simulink model "ducted_fan"  (R2014a)
settings: Solver=ode45  StartTime=0.0  StopTime=10.0  RelTol=1e-3
undefined symbols (not defined in the file): DiscIntNeverNeededParam, ST
libraries: simulink_extras x15
settings Model: Creator=stefa  LastModifiedBy=stefa

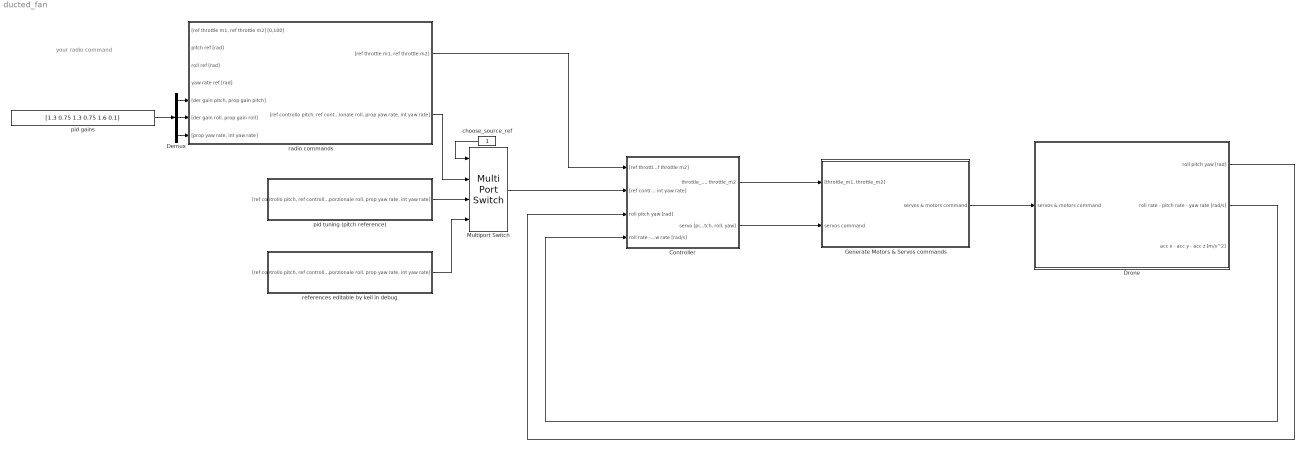
== system ducted_fan ==
  note: your radio command
  Controller : Subsystem
  Demux : Demux  Outputs=[2 2 2]
  Drone : Subsystem
  Generate Motors & Servos commands : Subsystem
  Multiport Switch : MultiPortSwitch
  choose_source_ref : Constant
  pid gains : Constant  Value=[1.3 0.75 1.3 0.75 1.6 0.1]
  pid tuning (pitch reference) : Subsystem
  radio commands : Subsystem
  references editable by keil in debug : Subsystem
  wires:
  Drone/1(roll pitch yaw [rad]) -> Controller/3(roll pitch yaw [rad])
  Drone/2(roll rate - pitch rate - yaw rate [rad/s]) -> Controller/4(roll rate - pitch rate - yaw rate [rad/s])
  Controller/2("servo [pitch, roll, yaw]") -> Generate Motors & Servos commands/2(servos command)
  Generate Motors & Servos commands/1(servos & motors command) -> Drone/1(servos & motors command)
  Controller/1("throttle_m1, throttle_m2") -> Generate Motors & Servos commands/1("[throttle_m1, throttle_m2]")
  choose_source_ref/1 -> Multiport Switch/1
  Multiport Switch/1 -> Controller/2("[ref controllo pitch, ref controllo roll, ref controllo yaw rate, guadagno derivativo pitch, guadagno proporzionale pitch, guadagno derivativo roll, guadagno proporzionale roll, prop yaw rate, int yaw rate]")
  radio commands/2("[ref controllo pitch, ref controllo roll, ref controllo yaw rate, guadagno derivativo pitch, guadagno proporzionale pitch, guadagno derivativo roll, guadagno proporzionale roll, prop yaw rate, int yaw rate]") -> Multiport Switch/2
  pid tuning (pitch reference)/1("[ref controllo pitch, ref controllo roll, ref controllo yaw rate, guadagno derivativo pitch, guadagno proporzionale pitch, guadagno derivativo roll, guadagno proporzionale roll, prop yaw rate, int yaw rate]") -> Multiport Switch/3
  references editable by keil in debug/1("[ref controllo pitch, ref controllo roll, ref controllo yaw rate, guadagno derivativo pitch, guadagno proporzionale pitch, guadagno derivativo roll, guadagno proporzionale roll, prop yaw rate, int yaw rate]") -> Multiport Switch/4
  radio commands/1("[ref throttle m1, ref throttle m2]") -> Controller/1("[ref throttle m1, ref throttle m2]")
  ? -> radio commands/1("[ref throttle m1, ref throttle m2] [0,100]")
  ? -> radio commands/2(pitch ref [rad])
  ? -> radio commands/3(roll ref [rad])
  ? -> radio commands/4(yaw rate ref [rad])
  Demux/2 -> radio commands/6("[der gain roll, prop gain roll]")
  Demux/1 -> radio commands/5("[der gain pitch, prop gain pitch]")
  Demux/3 -> radio commands/7("[prop yaw rate, int yaw rate]")
  pid gains/1 -> Demux/1

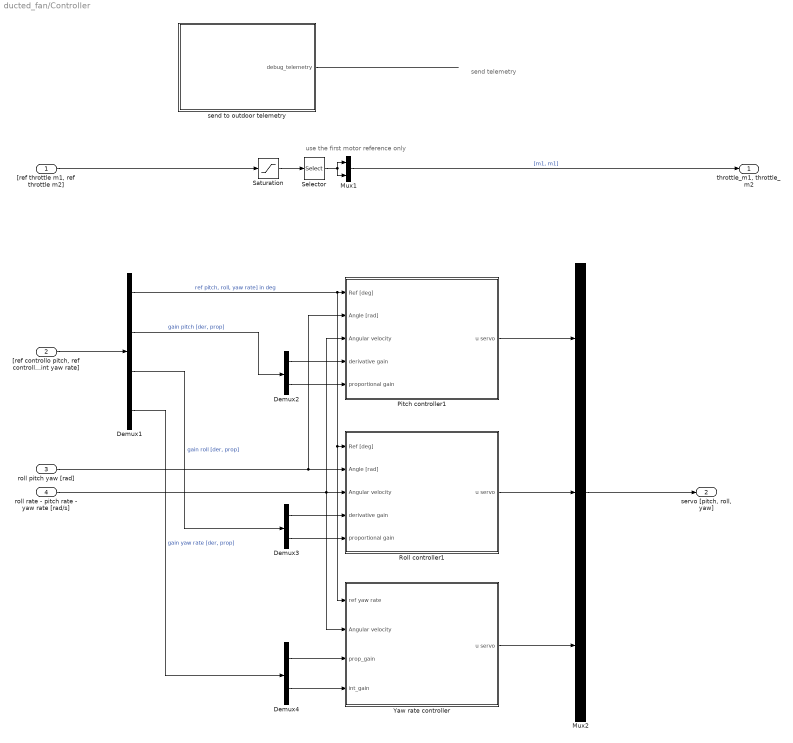
== system ducted_fan/Controller ==
  note: send telemetry
  note: use the first motor reference only
  "[ref throttle m1, ref throttle m2]" : Inport
  "[ref controllo pitch, ref controllo roll, ref controllo yaw rate, guadagno derivativo pitch, guadagno proporzionale pitch, guadagno derivativo roll, guadagno proporzionale roll, prop yaw rate, int yaw rate]" : Inport  Port=2
  roll pitch yaw [rad] : Inport  Port=3
  roll rate - pitch rate - yaw rate [rad/s] : Inport  Port=4
  Demux1 : Demux  Outputs=[3 2 2 2]
  Demux2 : Demux  Outputs=2
  Demux3 : Demux  Outputs=2
  Demux4 : Demux  Outputs=2
  Mux1 : Mux  Inputs=2
  Mux2 : Mux  Inputs=3
  Pitch controller1 : Subsystem
  Roll controller1 : Subsystem
  Saturation : Saturate  UpperLimit=100  LowerLimit=0
  Selector : Selector  InputPortWidth=2
  Yaw rate controller : Subsystem
  "send to outdoor telemetry " : Subsystem
  "throttle_m1, throttle_m2" : Outport
  "servo [pitch, roll, yaw]" : Outport  Port=2
  wires:
  Saturation/1 -> Selector/1
  Selector/1 -> Mux1/2, Mux1/1
  Mux1/1 -> "throttle_m1, throttle_m2"/1  "[m1, m1]"
  roll pitch yaw [rad]/1 -> Pitch controller1/2(Angle [rad]), Roll controller1/2(Angle [rad])
  roll rate - pitch rate - yaw rate [rad/s]/1 -> Pitch controller1/3(Angular velocity), Yaw rate controller/2(Angular velocity), Roll controller1/3(Angular velocity)
  Pitch controller1/1(u servo) -> Mux2/1
  Mux2/1 -> "servo [pitch, roll, yaw]"/1
  "[ref controllo pitch, ref controllo roll, ref controllo yaw rate, guadagno derivativo pitch, guadagno proporzionale pitch, guadagno derivativo roll, guadagno proporzionale roll, prop yaw rate, int yaw rate]"/1 -> Demux1/1
  Demux1/1 -> Yaw rate controller/1(ref yaw rate), Roll controller1/1(Ref [deg]), Pitch controller1/1(Ref [deg])  "ref pitch, roll, yaw rate] in deg"
  Roll controller1/1(u servo) -> Mux2/2
  Yaw rate controller/1(u servo) -> Mux2/3
  Demux1/2 -> Demux2/1  "gain pitch [der, prop]"
  Demux2/2 -> Pitch controller1/5(proportional gain)
  Demux2/1 -> Pitch controller1/4(derivative gain)
  Demux1/3 -> Demux3/1  "gain roll [der, prop]"
  Demux3/1 -> Roll controller1/4(derivative gain)
  Demux3/2 -> Roll controller1/5(proportional gain)
  Demux1/4 -> Demux4/1  "gain yaw rate [der, prop]"
  Demux4/1 -> Yaw rate controller/3(prop_gain)
  Demux4/2 -> Yaw rate controller/4(int_gain)
  "[ref throttle m1, ref throttle m2]"/1 -> Saturation/1
  "send to outdoor telemetry "/1(debug_telemetry) -> ?

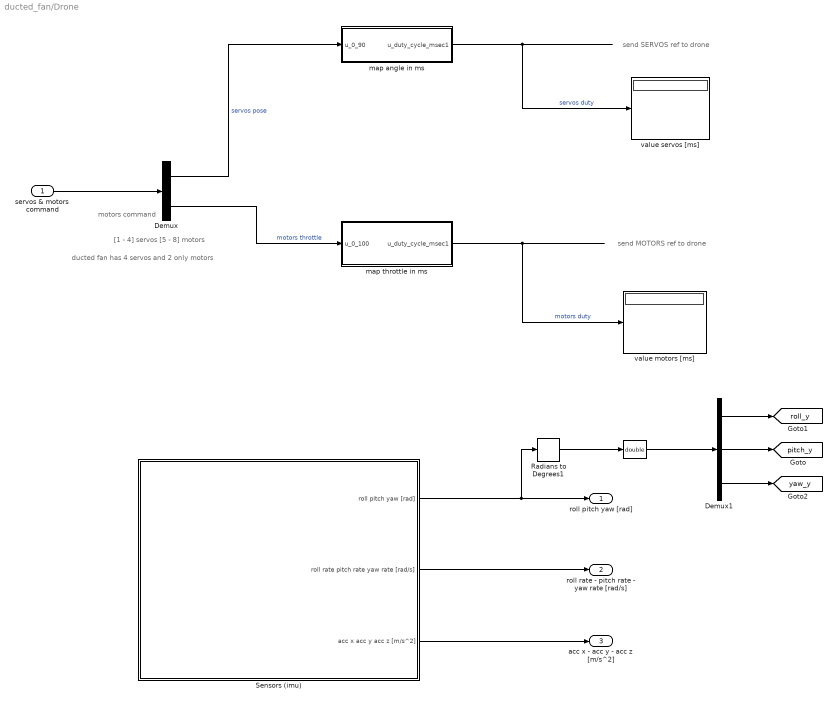
== system ducted_fan/Drone ==
  note: send SERVOS ref to drone
  note: ducted fan has 4 servos and 2 only motors
  note: [1 - 4] servos
      | [5 - 8] motors
  note: motors command
  note: send MOTORS ref to drone
  servos & motors command : Inport
  "  " : DataTypeConversion  OutDataTypeStr=double
  Demux : Demux  Outputs=[4 4]
  Demux1 : Demux  Outputs=3
  Radians to Degrees1 : simulink_extras/Transformations/Radians to Degrees
  Sensors (imu) : Subsystem
  map angle in ms : MATLAB Function  TreatAsAtomicUnit=on
  map throttle in ms : MATLAB Function  TreatAsAtomicUnit=on
  value motors [ms] : Display
  value servos [ms] : Display
  roll pitch yaw [rad] : Outport
  roll rate - pitch rate - yaw rate [rad/s] : Outport  Port=2
  acc x - acc y - acc z [m/s^2] : Outport  Port=3
  tag scope: pitch_y=global, roll_y=global, yaw_y=global
  wires:
  servos & motors command/1 -> Demux/1
  Demux/1 -> map angle in ms/1(u_0_90)  "servos pose"
  map throttle in ms/1(u_duty_cycle_msec1) -> value motors [ms]/1  "motors duty"
  map angle in ms/1(u_duty_cycle_msec1) -> value servos [ms]/1  "servos duty"
  Sensors (imu)/1(roll pitch yaw [rad]) -> Radians to Degrees1/1, roll pitch yaw [rad]/1
  Sensors (imu)/2(roll rate pitch rate yaw rate [rad/s]) -> roll rate - pitch rate - yaw rate [rad/s]/1
  Sensors (imu)/3(acc x acc y acc z [m/s^2]) -> acc x - acc y - acc z [m/s^2]/1
  Demux/2 -> map throttle in ms/1(u_0_100)  "motors throttle"
  Demux1/2 -> [pitch_y]
  Demux1/1 -> [roll_y]
  Radians to Degrees1/1 -> "  "/1
  "  "/1 -> Demux1/1
  Demux1/3 -> [yaw_y]

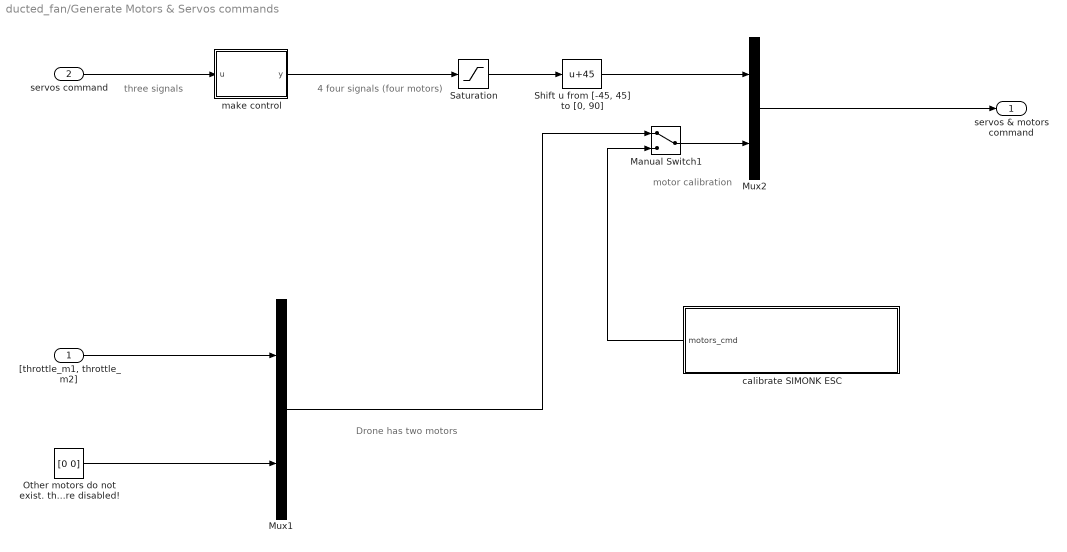
== system ducted_fan/Generate Motors & Servos commands ==
  note: 4 four signals (four motors)
  note: three signals
  note: Drone has two motors
  note: motor
      | calibration
  "[throttle_m1, throttle_m2]" : Inport
  servos command : Inport  Port=2
  Manual Switch1 : ManualSwitch
  Mux1 : Mux  Inputs=[2 2]
  Mux2 : Mux  Inputs=2
  Other motors do not exist. they are disabled! : Constant  Value=[0 0]
  Saturation : Saturate  UpperLimit=45  LowerLimit=-45
  "Shift u from [-45, 45] to [0, 90]" : Bias  Bias=45
  calibrate SIMONK ESC : Subsystem
  make control : MATLAB Function  TreatAsAtomicUnit=on
  servos & motors command : Outport
  wires:
  Mux2/1 -> servos & motors command/1
  Mux1/1 -> Manual Switch1/1
  calibrate SIMONK ESC/1(motors_cmd) -> Manual Switch1/2
  make control/1(y) -> Saturation/1
  Other motors do not exist. they are disabled!/1 -> Mux1/2
  Manual Switch1/1 -> Mux2/2
  servos command/1 -> make control/1(u)
  "[throttle_m1, throttle_m2]"/1 -> Mux1/1
  "Shift u from [-45, 45] to [0, 90]"/1 -> Mux2/1
  Saturation/1 -> "Shift u from [-45, 45] to [0, 90]"/1

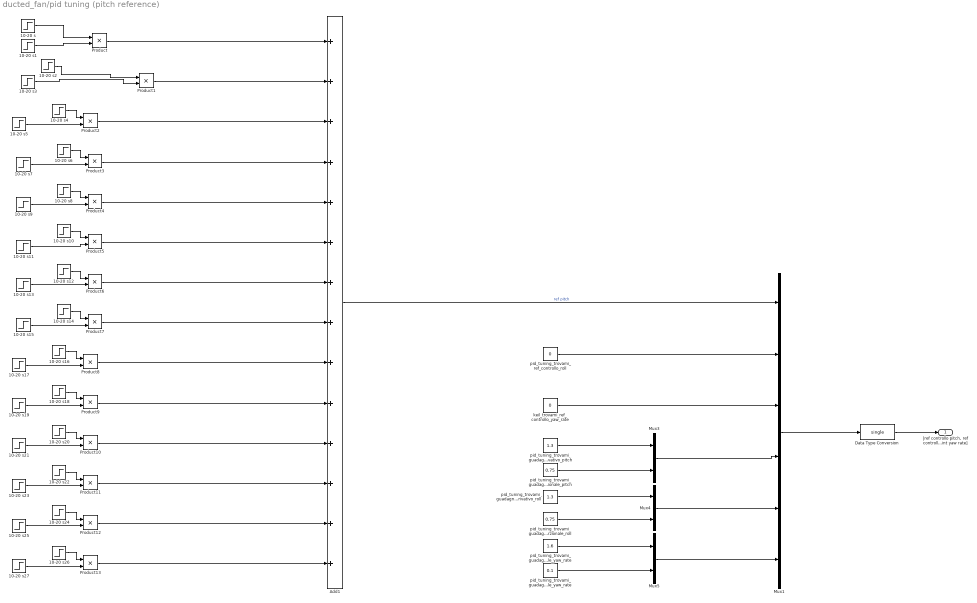
== system ducted_fan/pid tuning (pitch reference) ==
  10-20 s : Step  Time=20  After=10
  10-20 s1 : Step  Time=30  Before=1  After=0
  10-20 s10 : Step  Time=70  After=0
  10-20 s11 : Step  Time=80  Before=1  After=0
  10-20 s12 : Step  Time=80  After=-10
  10-20 s13 : Step  Time=90  Before=1  After=0
  10-20 s14 : Step  Time=90  After=0
  10-20 s15 : Step  Time=100  Before=1  After=0
  10-20 s16 : Step  Time=100  After=-20
  10-20 s17 : Step  Time=110  Before=1  After=0
  10-20 s18 : Step  Time=110  After=0
  10-20 s19 : Step  Time=120  Before=1  After=0
  10-20 s2 : Step  Time=30  After=0
  10-20 s20 : Step  Time=120  After=-30
  10-20 s21 : Step  Time=130  Before=1  After=0
  10-20 s22 : Step  Time=130  After=0
  10-20 s23 : Step  Time=140  Before=1  After=0
  10-20 s24 : Step  Time=140  After=40
  10-20 s25 : Step  Time=150  Before=1  After=0
  10-20 s26 : Step  Time=150  After=-40
  10-20 s27 : Step  Time=160  Before=1  After=0
  10-20 s3 : Step  Time=40  Before=1  After=0
  10-20 s4 : Step  Time=40  After=20
  10-20 s5 : Step  Time=50  Before=1  After=0
  10-20 s6 : Step  Time=50  After=0
  10-20 s7 : Step  Time=60  Before=1  After=0
  10-20 s8 : Step  Time=60  After=30
  10-20 s9 : Step  Time=70  Before=1  After=0
  Add1 : Sum  Inputs=++++++++++++++
  Data Type Conversion : DataTypeConversion  OutDataTypeStr=single
  Mux1 : Mux  Inputs=6
  Mux3 : Mux  Inputs=2
  Mux4 : Mux  Inputs=2
  Mux5 : Mux  Inputs=2
  Product{,1..13} (14 alike) : Product
  keil_trovami_ref_controllo_yaw_rate : Constant  Value=0  OutDataTypeStr=double  SampleTime=-1
  pid_tuning_trovami_guadagno_derivativo_pitch : Constant  Value=1.3  SampleTime=-1
  pid_tuning_trovami_guadagno_derivativo_roll : Constant  Value=1.3  SampleTime=-1
  pid_tuning_trovami_guadagno_integrale_yaw_rate : Constant  Value=0.1  SampleTime=-1
  pid_tuning_trovami_guadagno_proporzionale_pitch : Constant  Value=0.75  SampleTime=-1
  pid_tuning_trovami_guadagno_proporzionale_roll : Constant  Value=0.75  SampleTime=-1
  pid_tuning_trovami_guadagno_proporzionale_yaw_rate : Constant  Value=1.6  SampleTime=-1
  pid_tuning_trovami_ref_controllo_roll : Constant  Value=0  SampleTime=-1
  "[ref controllo pitch, ref controllo roll, ref controllo yaw rate, guadagno derivativo pitch, guadagno proporzionale pitch, guadagno derivativo roll, guadagno proporzionale roll, prop yaw rate, int yaw rate]" : Outport
  wires:
  Mux1/1 -> Data Type Conversion/1
  pid_tuning_trovami_ref_controllo_roll/1 -> Mux1/2
  10-20 s/1 -> Product/1
  Product/1 -> Add1/1
  10-20 s1/1 -> Product/2
  10-20 s2/1 -> Product1/1
  Product1/1 -> Add1/2
  10-20 s3/1 -> Product1/2
  10-20 s4/1 -> Product2/1
  Product2/1 -> Add1/3
  10-20 s5/1 -> Product2/2
  10-20 s6/1 -> Product3/1
  10-20 s7/1 -> Product3/2
  Product3/1 -> Add1/4
  10-20 s8/1 -> Product4/1
  10-20 s9/1 -> Product4/2
  Product4/1 -> Add1/5
  10-20 s10/1 -> Product5/1
  10-20 s11/1 -> Product5/2
  Product5/1 -> Add1/6
  10-20 s12/1 -> Product6/1
  10-20 s13/1 -> Product6/2
  Product6/1 -> Add1/7
  10-20 s14/1 -> Product7/1
  10-20 s15/1 -> Product7/2
  Product7/1 -> Add1/8
  10-20 s16/1 -> Product8/1
  10-20 s17/1 -> Product8/2
  Product8/1 -> Add1/9
  10-20 s18/1 -> Product9/1
  10-20 s19/1 -> Product9/2
  Product9/1 -> Add1/10
  10-20 s20/1 -> Product10/1
  10-20 s21/1 -> Product10/2
  Product10/1 -> Add1/11
  10-20 s22/1 -> Product11/1
  10-20 s23/1 -> Product11/2
  Product11/1 -> Add1/12
  10-20 s24/1 -> Product12/1
  10-20 s25/1 -> Product12/2
  Product12/1 -> Add1/13
  10-20 s26/1 -> Product13/1
  10-20 s27/1 -> Product13/2
  Product13/1 -> Add1/14
  Add1/1 -> Mux1/1  "ref pitch"
  Data Type Conversion/1 -> "[ref controllo pitch, ref controllo roll, ref controllo yaw rate, guadagno derivativo pitch, guadagno proporzionale pitch, guadagno derivativo roll, guadagno proporzionale roll, prop yaw rate, int yaw rate]"/1
  pid_tuning_trovami_guadagno_derivativo_pitch/1 -> Mux3/1
  pid_tuning_trovami_guadagno_derivativo_roll/1 -> Mux4/1
  pid_tuning_trovami_guadagno_proporzionale_pitch/1 -> Mux3/2
  Mux3/1 -> Mux1/4
  pid_tuning_trovami_guadagno_proporzionale_roll/1 -> Mux4/2
  Mux4/1 -> Mux1/5
  pid_tuning_trovami_guadagno_proporzionale_yaw_rate/1 -> Mux5/1
  pid_tuning_trovami_guadagno_integrale_yaw_rate/1 -> Mux5/2
  Mux5/1 -> Mux1/6
  keil_trovami_ref_controllo_yaw_rate/1 -> Mux1/3

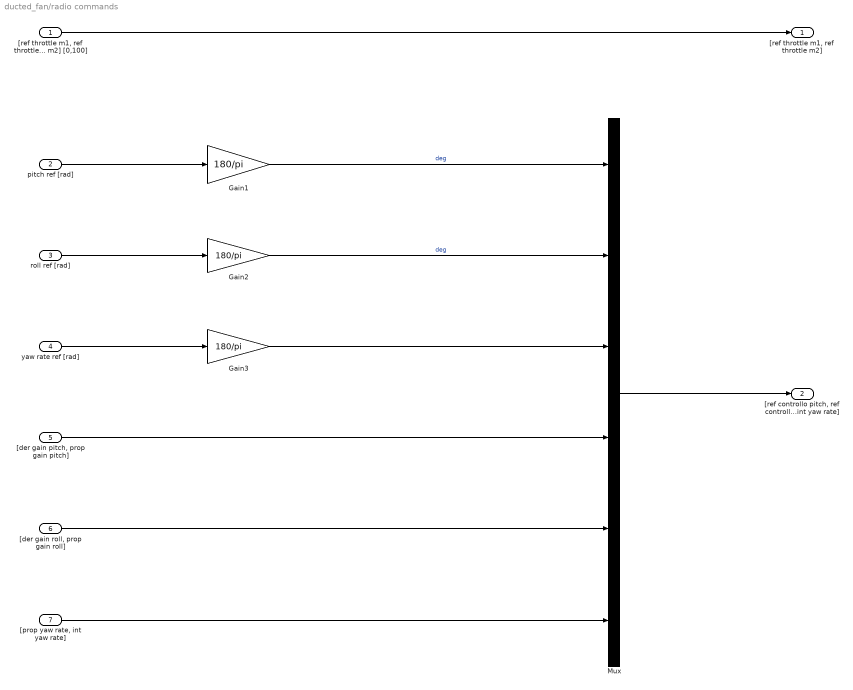
== system ducted_fan/radio commands ==
  "[ref throttle m1, ref throttle m2] [0,100]" : Inport
  pitch ref [rad] : Inport  Port=2
  roll ref [rad] : Inport  Port=3
  yaw rate ref [rad] : Inport  Port=4
  "[der gain pitch, prop gain pitch]" : Inport  Port=5
  "[der gain roll, prop gain roll]" : Inport  Port=6
  "[prop yaw rate, int yaw rate]" : Inport  Port=7
  Gain1 : Gain  Gain=180/pi
  Gain2 : Gain  Gain=180/pi
  Gain3 : Gain  Gain=180/pi
  Mux : Mux  Inputs=[1 1 1 2 2 2]
  "[ref throttle m1, ref throttle m2]" : Outport
  "[ref controllo pitch, ref controllo roll, ref controllo yaw rate, guadagno derivativo pitch, guadagno proporzionale pitch, guadagno derivativo roll, guadagno proporzionale roll, prop yaw rate, int yaw rate]" : Outport  Port=2
  wires:
  Mux/1 -> "[ref controllo pitch, ref controllo roll, ref controllo yaw rate, guadagno derivativo pitch, guadagno proporzionale pitch, guadagno derivativo roll, guadagno proporzionale roll, prop yaw rate, int yaw rate]"/1
  "[der gain pitch, prop gain pitch]"/1 -> Mux/4
  "[der gain roll, prop gain roll]"/1 -> Mux/5
  roll ref [rad]/1 -> Gain2/1
  Gain2/1 -> Mux/2  "deg"
  pitch ref [rad]/1 -> Gain1/1
  Gain1/1 -> Mux/1  "deg"
  "[prop yaw rate, int yaw rate]"/1 -> Mux/6
  yaw rate ref [rad]/1 -> Gain3/1
  Gain3/1 -> Mux/3
  "[ref throttle m1, ref throttle m2] [0,100]"/1 -> "[ref throttle m1, ref throttle m2]"/1

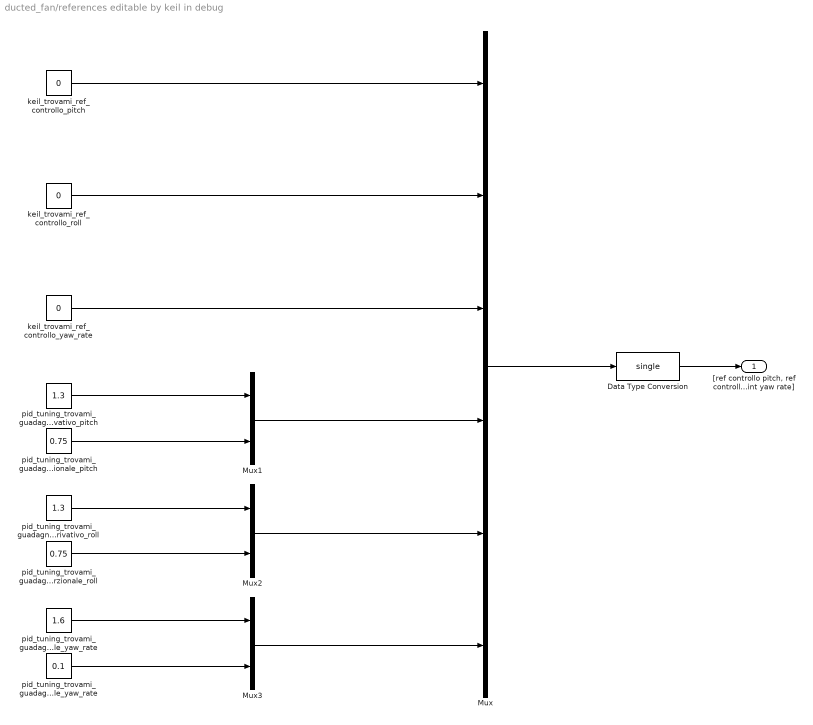
== system ducted_fan/references editable by keil in debug ==
  Data Type Conversion : DataTypeConversion  OutDataTypeStr=single
  Mux : Mux  Inputs=6
  Mux1 : Mux  Inputs=2
  Mux2 : Mux  Inputs=2
  Mux3 : Mux  Inputs=2
  keil_trovami_ref_controllo_pitch : Constant  Value=0  SampleTime=-1
  keil_trovami_ref_controllo_roll : Constant  Value=0  SampleTime=-1
  keil_trovami_ref_controllo_yaw_rate : Constant  Value=0  OutDataTypeStr=double  SampleTime=-1
  pid_tuning_trovami_guadagno_derivativo_pitch : Constant  Value=1.3  SampleTime=-1
  pid_tuning_trovami_guadagno_derivativo_roll : Constant  Value=1.3  SampleTime=-1
  pid_tuning_trovami_guadagno_integrale_yaw_rate : Constant  Value=0.1  SampleTime=-1
  pid_tuning_trovami_guadagno_proporzionale_pitch : Constant  Value=0.75  SampleTime=-1
  pid_tuning_trovami_guadagno_proporzionale_roll : Constant  Value=0.75  SampleTime=-1
  pid_tuning_trovami_guadagno_proporzionale_yaw_rate : Constant  Value=1.6  SampleTime=-1
  "[ref controllo pitch, ref controllo roll, ref controllo yaw rate, guadagno derivativo pitch, guadagno proporzionale pitch, guadagno derivativo roll, guadagno proporzionale roll, prop yaw rate, int yaw rate]" : Outport
  wires:
  Mux/1 -> Data Type Conversion/1
  keil_trovami_ref_controllo_pitch/1 -> Mux/1
  keil_trovami_ref_controllo_roll/1 -> Mux/2
  Data Type Conversion/1 -> "[ref controllo pitch, ref controllo roll, ref controllo yaw rate, guadagno derivativo pitch, guadagno proporzionale pitch, guadagno derivativo roll, guadagno proporzionale roll, prop yaw rate, int yaw rate]"/1
  pid_tuning_trovami_guadagno_derivativo_pitch/1 -> Mux1/1
  pid_tuning_trovami_guadagno_derivativo_roll/1 -> Mux2/1
  pid_tuning_trovami_guadagno_proporzionale_pitch/1 -> Mux1/2
  Mux1/1 -> Mux/4
  pid_tuning_trovami_guadagno_proporzionale_roll/1 -> Mux2/2
  Mux2/1 -> Mux/5
  pid_tuning_trovami_guadagno_proporzionale_yaw_rate/1 -> Mux3/1
  pid_tuning_trovami_guadagno_integrale_yaw_rate/1 -> Mux3/2
  Mux3/1 -> Mux/6
  keil_trovami_ref_controllo_yaw_rate/1 -> Mux/3

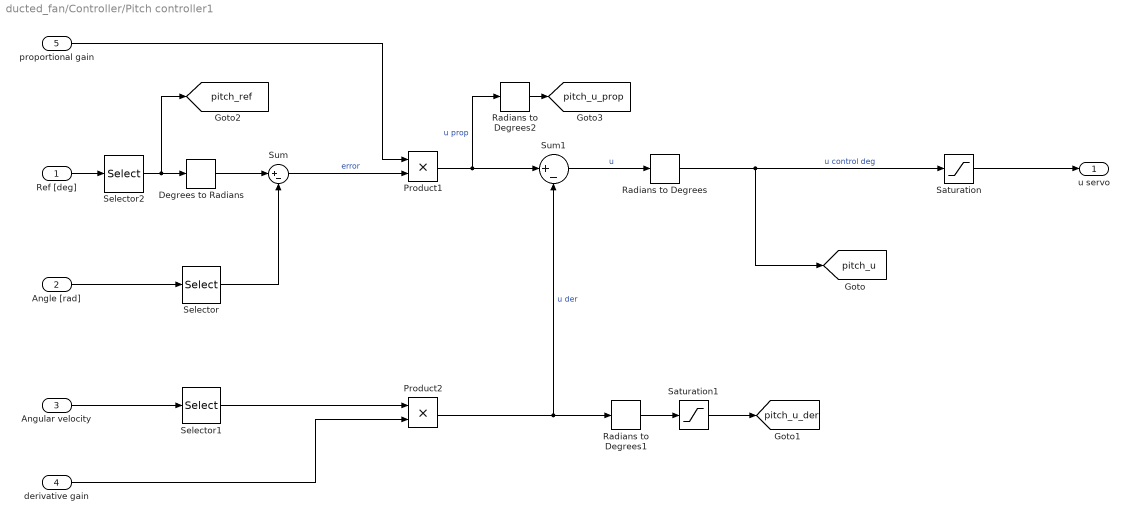
== system ducted_fan/Controller/Pitch controller1 ==
  Ref [deg] : Inport
  Angle [rad] : Inport  Port=2
  Angular velocity : Inport  Port=3
  derivative gain : Inport  Port=4
  proportional gain : Inport  Port=5
  Degrees to Radians : simulink_extras/Transformations/Degrees to Radians
  Product1 : Product
  Product2 : Product
  Radians to Degrees : simulink_extras/Transformations/Radians to Degrees
  Radians to Degrees1 : simulink_extras/Transformations/Radians to Degrees
  Radians to Degrees2 : simulink_extras/Transformations/Radians to Degrees
  Saturation : Saturate  UpperLimit=45  LowerLimit=-45
  Saturation1 : Saturate  UpperLimit=100  LowerLimit=-100
  Selector : Selector  InputPortWidth=3  Indices=2
  Selector1 : Selector  InputPortWidth=3  Indices=2
  Selector2 : Selector  InputPortWidth=3
  Sum : Sum  Inputs=|+-
  Sum1 : Sum  Inputs=|+-
  u servo : Outport
  tag scope: pitch_ref=global, pitch_u=global, pitch_u_der=global, pitch_u_prop=global
  wires:
  Angle [rad]/1 -> Selector/1
  Selector/1 -> Sum/2
  Product1/1 -> Radians to Degrees2/1, Sum1/1  "u prop"
  Angular velocity/1 -> Selector1/1
  Selector1/1 -> Product2/1
  Sum1/1 -> Radians to Degrees/1  "u"
  Radians to Degrees/1 -> Saturation/1, [pitch_u]  "u control deg"
  Degrees to Radians/1 -> Sum/1
  proportional gain/1 -> Product1/1
  derivative gain/1 -> Product2/2
  Sum/1 -> Product1/2  "error"
  Product2/1 -> Sum1/2, Radians to Degrees1/1  "u der"
  Radians to Degrees1/1 -> Saturation1/1
  Radians to Degrees2/1 -> [pitch_u_prop]
  Saturation1/1 -> [pitch_u_der]
  Saturation/1 -> u servo/1
  Ref [deg]/1 -> Selector2/1
  Selector2/1 -> [pitch_ref], Degrees to Radians/1

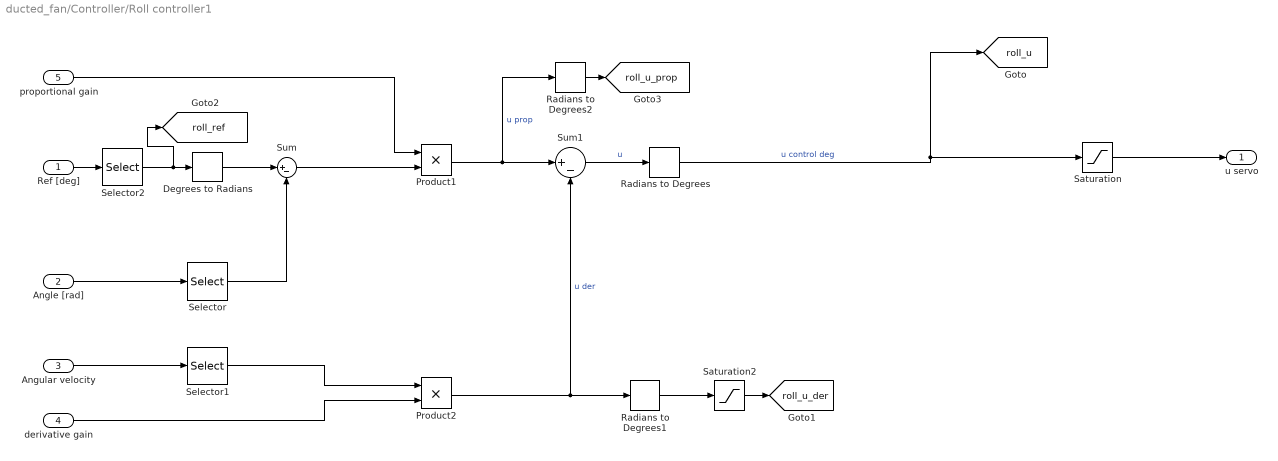
== system ducted_fan/Controller/Roll controller1 ==
  Ref [deg] : Inport
  Angle [rad] : Inport  Port=2
  Angular velocity : Inport  Port=3
  derivative gain : Inport  Port=4
  proportional gain : Inport  Port=5
  Degrees to Radians : simulink_extras/Transformations/Degrees to Radians
  Product1 : Product
  Product2 : Product
  Radians to Degrees : simulink_extras/Transformations/Radians to Degrees
  Radians to Degrees1 : simulink_extras/Transformations/Radians to Degrees
  Radians to Degrees2 : simulink_extras/Transformations/Radians to Degrees
  Saturation : Saturate  UpperLimit=45  LowerLimit=-45
  Saturation2 : Saturate  UpperLimit=100  LowerLimit=-100
  Selector : Selector  InputPortWidth=3
  Selector1 : Selector  InputPortWidth=3
  Selector2 : Selector  InputPortWidth=3  Indices=2
  Sum : Sum  Inputs=|+-
  Sum1 : Sum  Inputs=|+-
  u servo : Outport
  tag scope: roll_ref=global, roll_u=global, roll_u_der=global, roll_u_prop=global
  wires:
  Angle [rad]/1 -> Selector/1
  Selector/1 -> Sum/2
  Product1/1 -> Radians to Degrees2/1, Sum1/1  "u prop"
  Angular velocity/1 -> Selector1/1
  Selector1/1 -> Product2/1
  Sum1/1 -> Radians to Degrees/1  "u"
  Radians to Degrees/1 -> Saturation/1, [roll_u]  "u control deg"
  Degrees to Radians/1 -> Sum/1
  proportional gain/1 -> Product1/1
  derivative gain/1 -> Product2/2
  Ref [deg]/1 -> Selector2/1
  Sum/1 -> Product1/2
  Product2/1 -> Sum1/2, Radians to Degrees1/1  "u der"
  Radians to Degrees1/1 -> Saturation2/1
  Radians to Degrees2/1 -> [roll_u_prop]
  Saturation2/1 -> [roll_u_der]
  Saturation/1 -> u servo/1
  Selector2/1 -> [roll_ref], Degrees to Radians/1

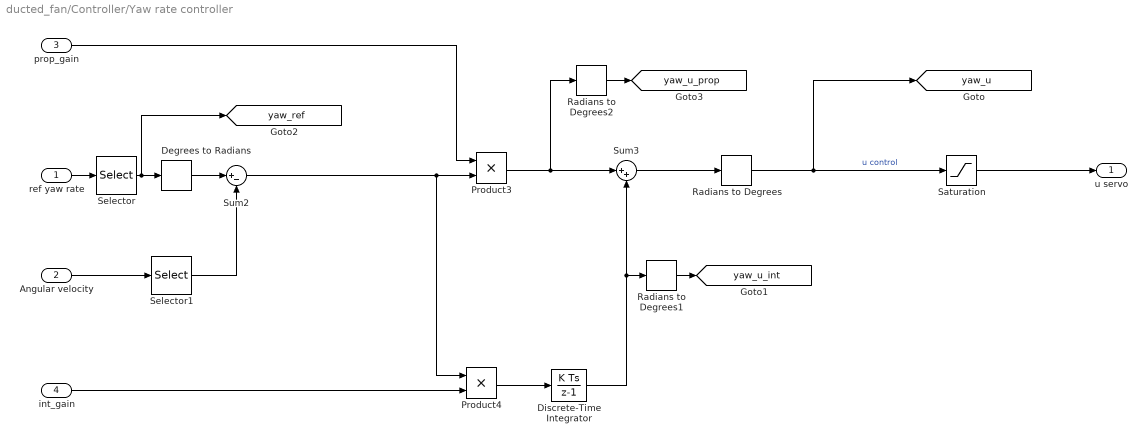
== system ducted_fan/Controller/Yaw rate controller ==
  ref yaw rate : Inport
  Angular velocity : Inport  Port=2
  prop_gain : Inport  Port=3
  int_gain : Inport  Port=4
  Degrees to Radians : simulink_extras/Transformations/Degrees to Radians
  Discrete-Time Integrator : DiscreteIntegrator  SampleTime=0.005  ICPrevOutput=DiscIntNeverNeededParam  ICPrevScaledInput=DiscIntNeverNeededParam
  Product3 : Product  RndMeth=Zero
  Product4 : Product  RndMeth=Zero
  Radians to Degrees : simulink_extras/Transformations/Radians to Degrees
  Radians to Degrees1 : simulink_extras/Transformations/Radians to Degrees
  Radians to Degrees2 : simulink_extras/Transformations/Radians to Degrees
  Saturation : Saturate  UpperLimit=45  LowerLimit=-45
  Selector : Selector  InputPortWidth=3  Indices=3
  Selector1 : Selector  InputPortWidth=3  Indices=3
  Sum2 : Sum  Inputs=|+-
  Sum3 : Sum  Inputs=|++
  u servo : Outport
  tag scope: yaw_ref=global, yaw_u=global, yaw_u_int=global, yaw_u_prop=global
  wires:
  Angular velocity/1 -> Selector1/1
  Radians to Degrees/1 -> [yaw_u], Saturation/1  "u control"
  Saturation/1 -> u servo/1
  Sum2/1 -> Product3/2, Product4/1
  ref yaw rate/1 -> Selector/1
  Sum3/1 -> Radians to Degrees/1
  Selector1/1 -> Sum2/2
  Product3/1 -> Radians to Degrees2/1, Sum3/1
  Product4/1 -> Discrete-Time Integrator/1
  Discrete-Time Integrator/1 -> Radians to Degrees1/1, Sum3/2
  prop_gain/1 -> Product3/1
  Radians to Degrees1/1 -> [yaw_u_int]
  Radians to Degrees2/1 -> [yaw_u_prop]
  Degrees to Radians/1 -> Sum2/1
  int_gain/1 -> Product4/2
  Selector/1 -> [yaw_ref], Degrees to Radians/1

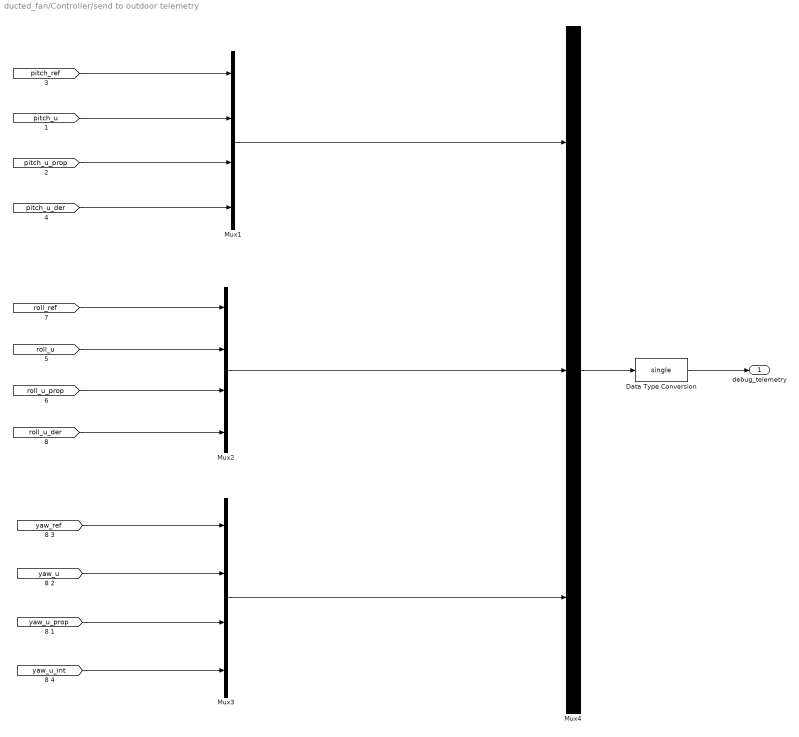
== system ducted_fan/Controller/send to outdoor telemetry  ==
  Data Type Conversion : DataTypeConversion  OutDataTypeStr=single
  Mux1 : Mux  Inputs=[1,1,1,1]
  Mux2 : Mux  Inputs=[1,1,1,1]
  Mux3 : Mux
  Mux4 : Mux  Inputs=[4 4 4]
  debug_telemetry : Outport  OutputWhenDisabled=reset  InitialOutput=0
  wires:
  [pitch_u_prop] -> Mux1/3
  [pitch_u_der] -> Mux1/4
  [roll_u] -> Mux2/2
  [roll_u_prop] -> Mux2/3
  [roll_u_der] -> Mux2/4
  [pitch_u] -> Mux1/2
  Mux2/1 -> Mux4/2
  Mux1/1 -> Mux4/1
  Mux3/1 -> Mux4/3
  [yaw_u] -> Mux3/2
  [yaw_ref] -> Mux3/1
  Mux4/1 -> Data Type Conversion/1
  Data Type Conversion/1 -> debug_telemetry/1
  [yaw_u_int] -> Mux3/4
  [yaw_u_prop] -> Mux3/3
  [pitch_ref] -> Mux1/1
  [roll_ref] -> Mux2/1

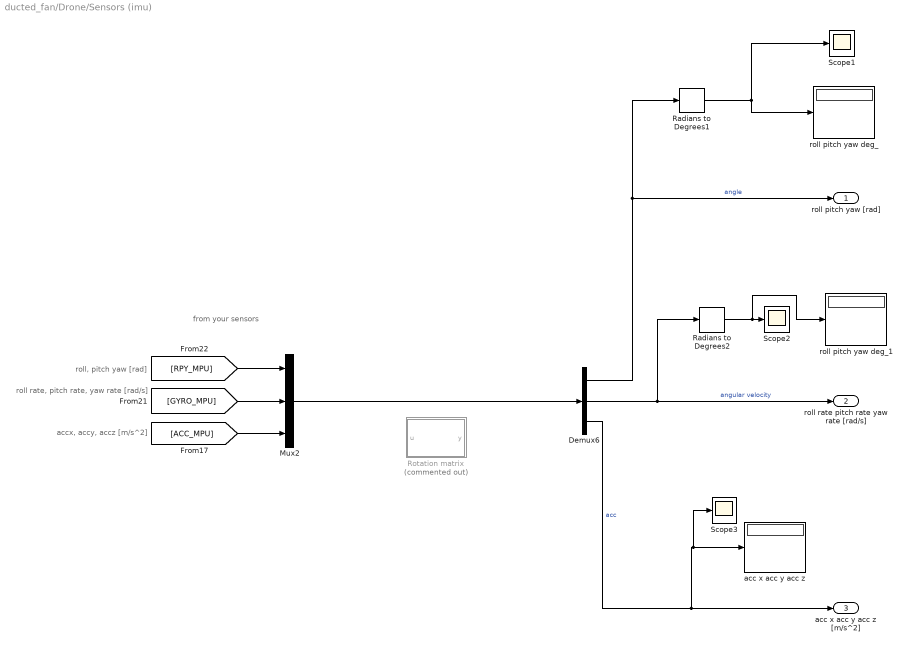
== system ducted_fan/Drone/Sensors (imu) ==
  note: accx, accy, accz [m/s^2]
  note: roll rate, pitch rate, yaw rate [rad/s]
  note: roll, pitch yaw [rad]
  note: from your sensors
  Demux6 : Demux  Outputs=[3 3 3]
  Mux2 : Mux  Inputs=[3 3 3 ]
  Radians to Degrees1 : simulink_extras/Transformations/Radians to Degrees
  Radians to Degrees2 : simulink_extras/Transformations/Radians to Degrees
  Rotation matrix : MATLAB Function  Commented=on  TreatAsAtomicUnit=on
  Scope1 : Scope
      settings: TickLabels=on  ShowLegends=on  YMin=-35  YMax=65  SaveName=ScopeData4
  Scope2 : Scope
      settings: TickLabels=on  ShowLegends=on  YMin=-35  YMax=65
  Scope3 : Scope
      settings: TickLabels=on  ShowLegends=on  YMin=-35  YMax=65  SaveName=ScopeData3
  acc x acc y acc z : Display
  roll pitch yaw deg_ : Display
  roll pitch yaw deg_1 : Display
  roll pitch yaw [rad] : Outport
  roll rate pitch rate yaw rate [rad/s] : Outport  Port=2
  acc x acc y acc z [m/s^2] : Outport  Port=3
  wires:
  Demux6/3 -> Scope3/1, acc x acc y acc z/1, acc x acc y acc z [m/s^2]/1  "acc"
  Demux6/1 -> roll pitch yaw [rad]/1, Radians to Degrees1/1  "angle"
  [RPY_MPU] -> Mux2/1
  [GYRO_MPU] -> Mux2/2
  [ACC_MPU] -> Mux2/3
  Radians to Degrees1/1 -> roll pitch yaw deg_/1, Scope1/1
  Demux6/2 -> roll rate pitch rate yaw rate [rad/s]/1, Radians to Degrees2/1  "angular velocity"
  Radians to Degrees2/1 -> roll pitch yaw deg_1/1, Scope2/1
  Mux2/1 -> Demux6/1

== system ducted_fan/Generate Motors & Servos commands/calibrate SIMONK ESC ==
  Product : Product  RndMeth=Zero
  Saturation : Saturate  UpperLimit=99  LowerLimit=0
  Sum : Sum  Inputs=|++
  Sum1 : Sum  Inputs=|++
  Sum2 : Sum  Inputs=|++
  calibrate Step : Step  Time=10  Before=[100 100 100 100]-1  After=[0 0 0 0]  SampleTime=ST  ZeroCross=off
  discrete time RAMP : Subsystem  mask{slope=10, start=30, X0=[0 0 0 0], ST_ramp=ST}
      mask prompts: start "start time"; X0 "initial output"; ST_ramp "sample time"
  disnable motors : Step  Time=60  After=-1  SampleTime=ST  ZeroCross=off
  enable motors cmd : Step  Time=20  SampleTime=ST  ZeroCross=off
  min speed : Constant  Value=[1 1 1 1]
  motors_cmd : Outport
  wires:
  Sum2/1 -> Product/1
  disnable motors/1 -> Sum2/2
  enable motors cmd/1 -> Sum2/1
  Saturation/1 -> Sum1/2
  Sum1/1 -> Product/2
  min speed/1 -> Sum1/1
  Product/1 -> Sum/2
  calibrate Step/1 -> Sum/1
  Sum/1 -> motors_cmd/1
  discrete time RAMP/1(y) -> Saturation/1

== system ducted_fan/Generate Motors & Servos commands/calibrate SIMONK ESC/discrete time RAMP ==
  Constant : Constant  DisableCoverage=on  Value=start  OutDataTypeStr=Inherit: Inherit via back propagation  SampleTime=ST
  Constant1 : Constant  DisableCoverage=on  Value=X0  OutDataTypeStr=Inherit: Inherit via back propagation  SampleTime=ST
  Digital Clock : DigitalClock  SampleTime=ST
  Output : Sum  Inputs=|++  SaturateOnIntegerOverflow=on  InputSameDT=on  OutDataTypeStr=Inherit: Same as first input
  Product1 : Product  DisableCoverage=on  SaturateOnIntegerOverflow=on  InputSameDT=on  OutDataTypeStr=Inherit: Same as first input
  Step : Step  DisableCoverage=on  Time=start  After=slope  SampleTime=ST  ZeroCross=off
  Sum3 : Sum  DisableCoverage=on  Inputs=|+-  SaturateOnIntegerOverflow=on  InputSameDT=on  OutDataTypeStr=Inherit: Same as first input
  y : Outport
  wires:
  Step/1 -> Product1/1
  Product1/1 -> Output/1
  Constant1/1 -> Output/2
  Output/1 -> y/1
  Sum3/1 -> Product1/2
  Constant/1 -> Sum3/2
  Digital Clock/1 -> Sum3/1

== matlab function ducted_fan/Drone/map angle in ms ==
  data: u_0_90 input; u_duty_cycle_msec1 output
function u_duty_cycle_msec1 = fcn(u_0_90)

N = 4;      % 4 servos

pwm_min = [1.050 0.8 1.0 0.9];          %msec
pwm_max = [1.810 1.5 1.9 1.6];          %msec

pwm_average = [1.42 1.15 1.5 1.23];     %msec

pwm_range_0_to_45 = pwm_average - pwm_min;
pwm_range_45_to_90 = pwm_max - pwm_average;

u_duty_cycle_msec1 = zeros(1,4);


%u_duty_cycle_msec1(1) = (pwm_min(1) + (u_0_90(1)/90.0) * pwm_range(1));

for i=1:N
    if u_0_90(i) <= 45
        u_duty_cycle_msec1(i) = pwm_min(i) + u_0_90(i) * (pwm_range_0_to_45(i) / 45);
    else
        u_duty_cycle_msec1(i) = pwm_average(i) - pwm_range_45_to_90(i) + u_0_90(i) * (pwm_range_45_to_90(i) / 45);
    end
end


%u_duty_cycle_msec1(2) = (pwm_min(2) + (u_0_90(2)/90.0) * pwm_range(2));
%u_duty_cycle_msec1(3) = (pwm_min(3) + (u_0_90(3)/90.0) * pwm_range);

%if u_0_90(3) <= 45
%    u_duty_cycle_msec1(3) = 0.9 + u_0_90(3)*(0.4/45);
%else
%    u_duty_cycle_msec1(3) = (pwm_min(3) + (u_0_90(3)/90.0) * pwm_range(3));
%end
%u_duty_cycle_msec1(4) = (pwm_min(4) + (u_0_90(4)/90.0) * pwm_range(4));


end

== matlab function ducted_fan/Drone/map throttle in ms ==
  data: u_0_100 input; u_duty_cycle_msec1 output
function u_duty_cycle_msec1 = fcn(u_0_100)
%#codegen
N = 2;

%define values for 0, 1, and range 100
pwm_min_m1 = .900; %msec
pwm_max_m1 = 1.750; %msec

pwm_min_m2 = .900; %msec
pwm_max_m2 = 1.990; %msec

pwm_range_m1 = pwm_max_m1 - pwm_min_m1;
pwm_range_m2 = pwm_max_m2 - pwm_min_m2;

u_duty_cycle_msec1 = zeros(1,4);            % force N=4


u_duty_cycle_msec1(1) = (pwm_min_m1+(u_0_100(1)/100.0)*pwm_range_m1);
u_duty_cycle_msec1(2) = (pwm_min_m2+(u_0_100(2)/100.0)*pwm_range_m2);

%This motor do not exist, just for compatibility
u_duty_cycle_msec1(3) = 0;
u_duty_cycle_msec1(4) = 0;

end

== matlab function ducted_fan/Generate Motors & Servos commands/make control ==
  data: u input; y output
function y = fcn(u)
%#codegen
%
% ducted fan has 4 servos
% by the symmetry we obtained the four u 
% u(1) -> pitch control (motors 1 and 3)
% u(2) -> roll control  (motors 2 and 4)
% u(3) -> yaw control   (motors 1 2 3 and 4)

% motors are represented by "@"
%      M1
%       ____
%     / @|  \
%    /   |   \
%   /    |   @\  M2
%  (=====o=====) 
%M4 @    |    /
%    \   |   /
%     \ _|@ /
%          M3


% yaw signal control is added to other signals control
% u = [-45, +45]

pose_m1 = - u(1) + u(3);
pose_m2 = u(2) + u(3);
pose_m3 = u(1) + u(3);
pose_m4 = - u(2) + u(3);


y = [pose_m1, pose_m2, pose_m3, pose_m4]';

== matlab function ducted_fan/Drone/Sensors (imu)/Rotation matrix ==
  data: u input; y output
function y = fcn(u)
%#% Declaring var
    pose = [u(1) u(2) u(3)]';
    posedot = [u(4) u(5) u(6)]';
    acc = [u(7) u(8) u(9)]';
    y = zeros(1,9);
%  Ximu    
%   .   ^ Xdes
%    \45|
%     \ |
%       +---->Ydes
%      /
%     / 
%    ' Zimu


    %% Rotation matrixes
    %% rot y  =>  remove 45° offset
%  Ximu    
%       ^ Ximu = Xdes
%       |
%  Zimu |
%  <----+---->Ydes
%        

    alpha = (3/4)*pi;
    Ry = [cos(alpha) 0 sin(alpha); 0 1 0; -sin(alpha) 0 cos(alpha)];
    
    %% rot x  => we would ned coord
%       ^ Ximu = Xdes
%       |
%       |
%       +----> Yimu = Ydes
%  Zimu = Zdes  
    
    beta = pi/2;
    Rx = [1 0 0 ; 0 cos(beta) -sin(beta); 0 sin(beta) cos(beta)];    
    
    %% Current axes
    R = Rx'*Ry';
    
    pose_ned = R*pose; %+ [0 62 0]'*pi/180;
    posedot_ned = R*posedot; %+ [-2, 1, 5]'*pi/180;
    acc_ned = R*acc;
    
    y(1:3) = pose_ned;
    y(4:6) = posedot_ned;
    y(7:9) = acc_ned;
